simulink model "db_lim"  (R2024b)
settings: Solver=VariableStepAuto  StartTime=0.0  StopTime=100.0  RelTol=1e-3
values from neighbouring files (symbols this model uses):
  Gp_z = c2d(Gp,T_vz)    [main.m]
  P = [1, p1, p2, p3]    [dB_controller.m]    (also in main.m = P_nolimit)
  Q = [q0, q1, q2, q3]    [dB_controller.m]    (also in main.m = Q_nolimit)
settings Model: Creator=egoru  LastModifiedBy=tolst

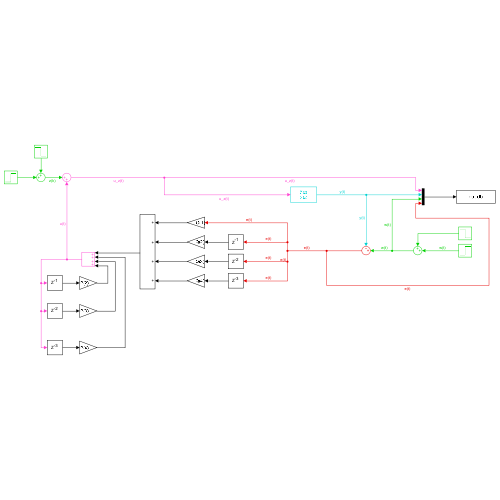
[thumbnail: Simulink's stored preview of the top-level diagram]
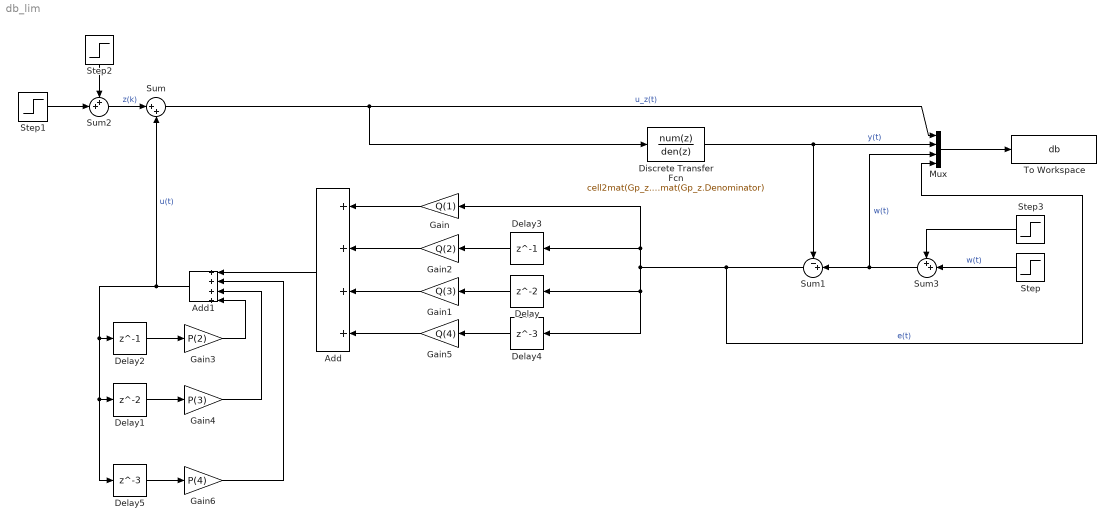
== system db_lim ==
  Add : Sum  Inputs=++++
  Add1 : Sum  Inputs=++++
  Delay : Delay
  Delay1 : Delay
  Delay2 : Delay  DelayLength=1
  Delay3 : Delay  DelayLength=1
  Delay4 : Delay  DelayLength=3
  Delay5 : Delay  DelayLength=3
  Discrete Transfer Fcn : DiscreteTransferFcn  Numerator=cell2mat(Gp_z.Numerator)  Denominator=cell2mat(Gp_z.Denominator)
  Gain : Gain  Gain=Q(1)
  Gain1 : Gain  Gain=Q(3)
  Gain2 : Gain  Gain=Q(2)
  Gain3 : Gain  Gain=P(2)
  Gain4 : Gain  Gain=P(3)
  Gain5 : Gain  Gain=Q(4)
  Gain6 : Gain  Gain=P(4)
  Mux : Mux
  Step : Step  Time=10  SampleTime=0
  Step1 : Step  Time=30  After=0.01  SampleTime=0
  Step2 : Step  Time=50  After=-0.01  SampleTime=0
  Step3 : Step  Time=70  After=-0.2  SampleTime=0
  Sum : Sum  Inputs=|++
  Sum1 : Sum  Inputs=-+|
  Sum2 : Sum  Inputs=++|
  Sum3 : Sum  Inputs=++|
  To Workspace : ToWorkspace  VariableName=db  SaveFormat=Timeseries  SampleTime=-1
  wires:
  Mux/1 -> To Workspace/1
  Discrete Transfer Fcn/1 -> Mux/2, Sum1/1  "y(t)"
  Sum1/1 -> Mux/4, Delay4/1, Delay/1, Delay3/1, Gain/1  "e(t)"
  Sum3/1 -> Mux/3, Sum1/2  "w(t)"
  Sum/1 -> Mux/1, Discrete Transfer Fcn/1  "u_z(t)"
  Add1/1 -> Delay5/1, Delay1/1, Delay2/1, Sum/2  "u(t)"
  Sum2/1 -> Sum/1  "z(k)"
  Add/1 -> Add1/1
  Gain2/1 -> Add/2
  Delay5/1 -> Gain6/1
  Gain6/1 -> Add1/2
  Gain/1 -> Add/1
  Gain5/1 -> Add/4
  Delay3/1 -> Gain2/1
  Delay2/1 -> Gain3/1
  Delay4/1 -> Gain5/1
  Delay/1 -> Gain1/1
  Delay1/1 -> Gain4/1
  Gain3/1 -> Add1/4
  Gain4/1 -> Add1/3
  Gain1/1 -> Add/3
  Step2/1 -> Sum2/1
  Step1/1 -> Sum2/2
  Step3/1 -> Sum3/1
  Step/1 -> Sum3/2  "w(t)"
